simulink model "first"  (R2016a)
settings: Solver=VariableStepAuto  StartTime=0.0  StopTime=10.0  RelTol=1e-3
settings Model: Creator=kypis  LastModifiedBy=kypis

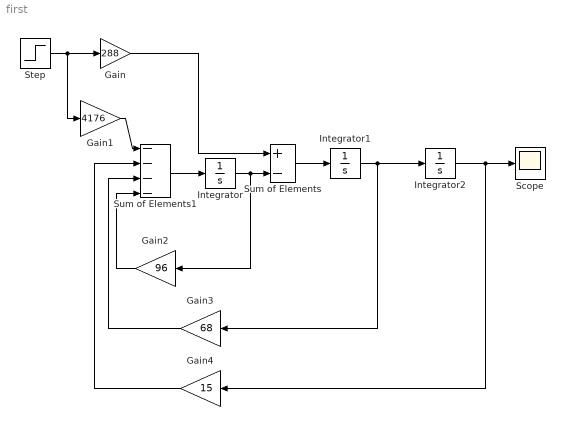
== system first ==
  Gain : Gain  Gain=288
  Gain1 : Gain  Gain=4176
  Gain2 : Gain  Gain=96
  Gain3 : Gain  Gain=68
  Gain4 : Gain  Gain=15
  Integrator : Integrator
  Integrator1 : Integrator
  Integrator2 : Integrator
  Scope : Scope
  Step : Step  Time=0  SampleTime=0
  Sum of Elements : Sum  Inputs=+-
  Sum of Elements1 : Sum  Inputs=----
  wires:
  Gain/1 -> Sum of Elements/1
  Step/1 -> Gain1/1, Gain/1
  Sum of Elements1/1 -> Integrator/1
  Gain1/1 -> Sum of Elements1/1
  Integrator/1 -> Gain2/1, Sum of Elements/2
  Integrator1/1 -> Gain3/1, Integrator2/1
  Sum of Elements/1 -> Integrator1/1
  Gain2/1 -> Sum of Elements1/4
  Gain3/1 -> Sum of Elements1/3
  Integrator2/1 -> Gain4/1, Scope/1
  Gain4/1 -> Sum of Elements1/2
